simulink library "A0EV_Lib1"  (Simulink 7.5)
settings: Solver=ode45  StartTime=0.0  StopTime=10.0  RelTol=1e-3
libraries: BaseOperationLib_Browser x6
settings Model: Creator=chenhongshuai  LastModifiedBy=guohongjiang

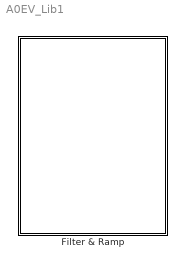
== system A0EV_Lib1 ==
  Filter & Ramp : Subsystem

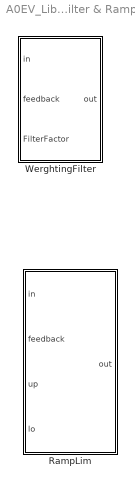
== system A0EV_Lib1/Filter & Ramp ==
  RampLim : Subsystem
      mask Display: plot([0.15 0.85],[0.5 0.5],[0.5 0.5],[0.15 0.85],[0.2 0.8],[0.2 0.8]);
  WerghtingFilter : Subsystem
      mask Display: plot([0.15 0.85],[0.5 0.5],[0.5 0.5],[0.15 0.85],[0.2 0.8],[0.2 0.8]);

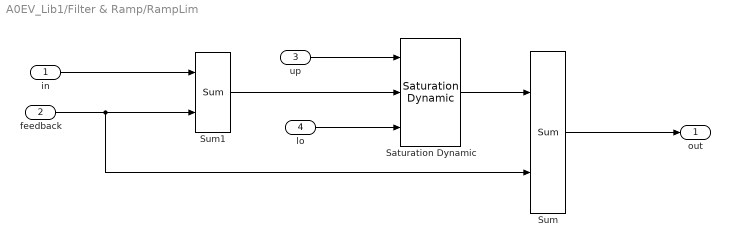
== system A0EV_Lib1/Filter & Ramp/RampLim ==
  in : Inport
  feedback : Inport  Port=2
  up : Inport  Port=3
  lo : Inport  Port=4
  Saturation Dynamic : BaseOperationLib_Browser/Discontinuities Unchanged/Saturation Dynamic  SystemSampleTime=-1  OutMin=[]  OutMax=[]  OutDataTypeStr=Inherit: Same as second input  OutDataType=fixdt(1, 16)  OutScaling=2^-10  DoSatur=off
  Sum : BaseOperationLib_Browser/Math Operations Changed/Sum  Inputs=++  InputSameDT=on  OutMin=[]  OutMax=[]  OutDataType=fixdt(1, 16)  OutScaling=2^0  SaturateOnIntegerOverflow=on
  Sum1 : BaseOperationLib_Browser/Math Operations Changed/Sum  Inputs=+-  InputSameDT=on  OutMin=[]  OutMax=[]  OutDataType=fixdt(1, 16)  OutScaling=2^0  SaturateOnIntegerOverflow=on
  out : Outport
  wires:
  Sum/1 -> out/1
  Sum1/1 -> Saturation Dynamic/2
  Saturation Dynamic/1 -> Sum/1
  in/1 -> Sum1/1
  up/1 -> Saturation Dynamic/1
  feedback/1 -> Sum/2, Sum1/2
  lo/1 -> Saturation Dynamic/3

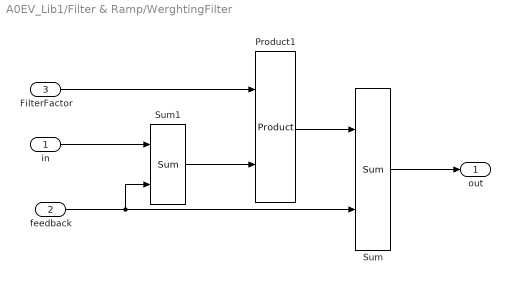
== system A0EV_Lib1/Filter & Ramp/WerghtingFilter ==
  in : Inport
  feedback : Inport  Port=2
  FilterFactor : Inport  Port=3
  Product1 : BaseOperationLib_Browser/Math Operations Changed/Product  Inputs=2  Multiplication=Element-wise(.*)  OutMin=[]  OutMax=[]  OutDataType=fixdt(1,16,0)  OutScaling=[]  OutDataTypeStr=Inherit: Inherit via back propagation  RndMeth=Zero  SaturateOnIntegerOverflow=on
  Sum : BaseOperationLib_Browser/Math Operations Changed/Sum  Inputs=++  InputSameDT=on  OutMin=[]  OutMax=[]  OutDataType=fixdt(1, 16)  OutScaling=2^0  SaturateOnIntegerOverflow=on
  Sum1 : BaseOperationLib_Browser/Math Operations Changed/Sum  Inputs=+-  InputSameDT=on  OutMin=[]  OutMax=[]  OutDataType=fixdt(1, 16)  OutScaling=2^0  SaturateOnIntegerOverflow=on
  out : Outport
  wires:
  Sum1/1 -> Product1/2
  Product1/1 -> Sum/1
  feedback/1 -> Sum1/2, Sum/2
  Sum/1 -> out/1
  in/1 -> Sum1/1
  FilterFactor/1 -> Product1/1
